simulink model "twopointcontrol"  (R2016b)
settings: Solver=FixedStepDiscrete  StartTime=0.0  StopTime=10.0  FixedStep=0.1  RelTol=1e-3
libraries: mbed_lib x5, mbed_targets_stm_nucleo_f446 x1, mbed_i2c_sensors x1
settings Model: Creator=Labor  LastModifiedBy=oh
settings DataIOCC: LimitDataPoints=on  SaveFormat=Array
settings OptimizationCC: LifeSpan=1
settings DebuggingCC: SFUnexpectedBacktrackingDiag=warning  SFNoUnconditionalDefaultTransitionDiag=warning  SFExecutionAtInitializationDiag=none
settings HardwareCC: ProdBitPerPointer=32  ProdBitPerSizeT=32  ProdBitPerPtrDiffT=32  ProdLargestAtomicInteger=Long  ProdLargestAtomicFloat=Double  ProdIntDivRoundTo=Undefined  ProdWordSize=32  ProdHWDeviceType=ARM Compatible->ARM Cortex
settings ModelReferenceCC: PropagateSignalLabelsOutOfModel=off
settings RTWCC: SystemTargetFile=mbed.tlc  TemplateMakefile=mbed.tmf  Description=Mbed Target (Embedded Target)  TargetLang=C++
settings CodeAppCC: IgnoreCustomStorageClasses=off
settings STFCustomTargetCC: TargetLibSuffix=.a  GenerateSampleERTMain=on  CombineOutputUpdateFcns=on  ERTCustomFileBanners=on  SupportContinuousTime=off  SupportNonInlinedSFcns=off  RemoveResetFunc=on  MATLABClassNameForMDSCustomization=Simulink.SoftwareTarget.ERTCustomization  GRTInterface=off  SystemTargetFile=mbed.tlc
settings ERTTargetCC: GenerateSampleERTMain=on  ParMdlRefBuildCompliant=off  CompOptLevelCompliant=off  ConcurrentExecutionCompliant=off  ERTFirstTimeCompliant=off  ModelStepFunctionPrototypeControlCompliant=off  CPPClassGenCompliant=off  UseToolchainInfoCompliant=off  ERTCustomFileTemplate=mbed_file_process.tlc  ConvertIfToSwitch=off  SuppressUnreachableDefaultCases=off
settings ConfigComp: CovMetricSettings=dw  CovHtmlReporting=on  CovSaveCumulativeToWorkspaceVar=on  CovSaveSingleToWorkspaceVar=on  CovExternalEMLEnable=off

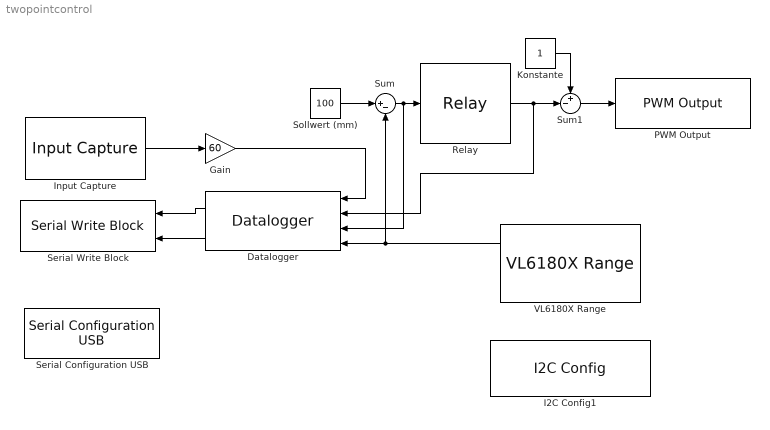
== system twopointcontrol ==
  Datalogger : mbed_lib/Utilities/Datalogger  TypeInputPorts={ 'single' 1 'single' 1 'double' 1 'single' 1 }  TypeOfInputs={'1*single' '1*single' '1*double' '1*single'}  BufferSize=100  errEn=off  SampleTime=-1
  Gain : Gain  Gain=60
  I2C Config1 : mbed_lib/Serial/I2C/I2C Config  Priority=0  I2CPort=1  Freq=100000  SDAPortName=B  SDAPinNumber=7  SCLPortName=B  SCLPinNumber=6
  Input Capture : mbed_targets_stm_nucleo_f446/Input Capture  TimerNumber=2  Frequency=100000  OutputMode=Frequency  Ti1Active=Rising  Ti1Port=A  Ti1Pin=0  Ti1Pupd=PullUp  Ti2Active=None  Ti2Port=A  Ti2Pin=0  Ti2Pupd=PullNone  Ti3Active=None  Ti3Port=A  Ti3Pin=0  Ti3Pupd=PullNone  Ti4Active=None  Ti4Port=A  Ti4Pin=0  Ti4Pupd=PullNone  SampleTime=-1
  "Konstante " : Constant  OutDataTypeStr=single
  PWM Output : mbed_lib/GPIO/PWM Output  PortName=A  PinNumber=0  Period=1000  SampleTime=-1
  Relay : Relay  OnSwitchValue=0  OffSwitchValue=0  OnOutputValue=0.97  OffOutputValue=0.94  OutDataTypeStr=single
  Serial Configuration USB : mbed_lib/Serial/UART/Serial Configuration USB  BaudRate=9600
  Serial Write Block : mbed_lib/Serial/UART/Serial Write Block  SerialPort=0  numData=on  SampleTime=-1
  Sollwert (mm) : Constant  Value=100
  Sum : Sum  Inputs=|+-
  Sum1 : Sum  Inputs=+-|
  VL6180X Range : mbed_i2c_sensors/VL6180X Range   i2cbus=1  SubAddress=29  PortName=A  PinNumber=1  lowtreshhold=0  hightreshhold=200  EnableError=off  SampleTime=-1
  wires:
  Sum/1 -> Datalogger/3, Relay/1
  Sollwert (mm)/1 -> Sum/1
  VL6180X Range/1 -> Sum/2, Datalogger/4
  Datalogger/1 -> Serial Write Block/1
  Datalogger/2 -> Serial Write Block/2
  Sum1/1 -> PWM Output/1
  Relay/1 -> Datalogger/2, Sum1/2
  "Konstante "/1 -> Sum1/1
  Input Capture/1 -> Gain/1
  Gain/1 -> Datalogger/1
